simulink model "D_N_Selector"  (R2021a)
settings: Solver=VariableStepAuto  StartTime=0.0  StopTime=10.0  RelTol=1e-3
settings Model: PacingRate=0.010000  Creator=shind  LastModifiedBy=shind

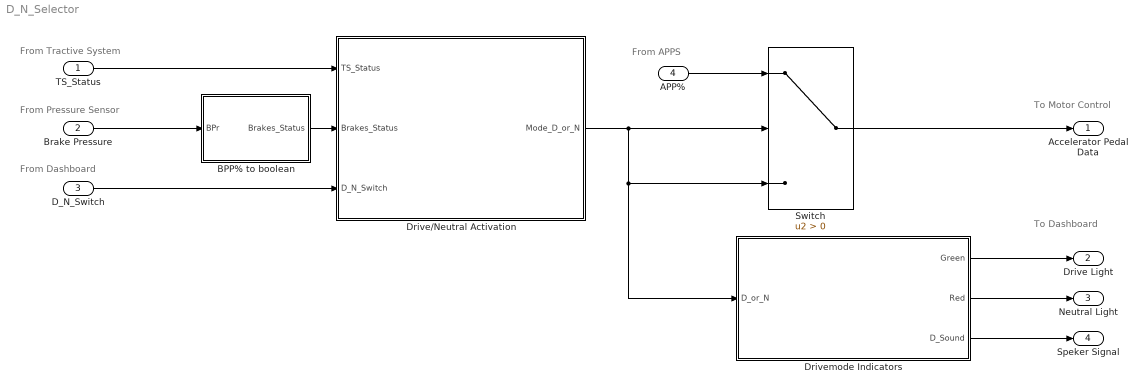
== system D_N_Selector ==
  note: From APPS
  note: From Pressure Sensor
  note: From Tractive System
  note: From Dashboard
  note: To Motor Control
  note: To Dashboard
  TS_Status : Inport
  Brake Pressure : Inport  Port=2
  D_N_Switch : Inport  Port=3
  APP% : Inport  Port=4
  BPP% to boolean : Stateflow chart  TreatAsAtomicUnit=on
  Drive/Neutral Activation : Stateflow chart  TreatAsAtomicUnit=on
  Drivemode Indicators : Stateflow chart  TreatAsAtomicUnit=on
  Switch : Switch  Criteria=u2 > Threshold
  Accelerator Pedal Data : Outport
  Drive Light : Outport  Port=2
  Neutral Light : Outport  Port=3
  Speker Signal : Outport  Port=4
  wires:
  TS_Status/1 -> Drive/Neutral Activation/1(TS_Status)
  Brake Pressure/1 -> BPP% to boolean/1(BPr)
  D_N_Switch/1 -> Drive/Neutral Activation/3(D_N_Switch)
  Drive/Neutral Activation/1(Mode_D_or_N) -> Switch/2, Drivemode Indicators/1(D_or_N), Switch/3
  APP%/1 -> Switch/1
  Switch/1 -> Accelerator Pedal Data/1
  Drivemode Indicators/1(Green) -> Drive Light/1
  Drivemode Indicators/2(Red) -> Neutral Light/1
  Drivemode Indicators/3(D_Sound) -> Speker Signal/1
  BPP% to boolean/1(Brakes_Status) -> Drive/Neutral Activation/2(Brakes_Status)

== stateflow chart D_N_Selector/Drivemode Indicators ==
  state Neutral
    entry:
    Red=1;
    Green=0;
  state Drive
    entry:
    Red=0;
    Green=1;
    state sound_start
      entry:
      D_Sound=1;
    state sound_stop
      entry:
      D_Sound=0;
    (default) -> sound_start
    sound_start -> sound_stop : after(2,sec)
  (default) -> Neutral
  Neutral -> Drive : [D_or_N==1]
  Drive -> Neutral : [D_or_N==0]
  data: D_or_N input; Green output; Red output; D_Sound output

== stateflow chart D_N_Selector/BPP% to boolean ==
  state Brakes_not_actuated
    entry:
    Brakes_Status==0;
  state Brakes_actuated
    entry:
    Brakes_Status==1;
  (default) -> Brakes_not_actuated
  Brakes_not_actuated -> Brakes_actuated : [BPr>20]
  Brakes_actuated -> Brakes_not_actuated : [BPr<20]
  data: BPr input; Brakes_Status output =00

== stateflow chart D_N_Selector/Drive//Neutral Activation ==
  state Neutral
    entry:
    Mode_D_or_N=0;
  state Consistant_action_check_for_D
  state Drive
    entry:
    Mode_D_or_N=1;
  state Consistant_action_check_for_N
  (default) -> Neutral
  Neutral -> Consistant_action_check_for_D : [Brakes_Status==1 && TS_Status==1 && D_N_Switch==1]
  Consistant_action_check_for_D -> Drive [order 2] : after(1,sec)
  Consistant_action_check_for_D -> Neutral [order 1] : [Brakes_Status==0 || TS_Status==0 || D_N_Switch==0]
  Drive -> Neutral [order 1] : [TS_Status==0]
  Drive -> Consistant_action_check_for_N [order 2] : [Brakes_Status==1 && D_N_Switch==1]
  Consistant_action_check_for_N -> Neutral [order 2] : after(500,msec)
  Consistant_action_check_for_N -> Drive [order 1] : [Brakes_Status==0 || D_N_Switch==0]
  data: TS_Status input; Brakes_Status input; D_N_Switch input; Mode_D_or_N output
